simulink model "propeller_sim"  (R2022a)
settings: Solver=VariableStepAuto  StartTime=0.0  StopTime=10.0  MaxStep=0.02  RelTol=1e-3
values from neighbouring files (symbols this model uses):
  b = 1    [class8_PropellerPendulum.m]    (also in class8_PropellerPendulum_Euler.m = 0.1; class8_PropellerPendulum_ode45.m; epsac.m = 0.1; propeller.m = Par(4))
  g = 9.8    [class8_PropellerPendulum.m]    (also in class8_PropellerPendulum_Euler.m = 9.81; class8_PropellerPendulum_ode45.m; epsac.m = 9.81; propeller.m = Par(5))
  h = 0.5    [class8_PropellerPendulum.m]    (also in class8_PropellerPendulum_Euler.m; class8_PropellerPendulum_ode45.m; epsac.m; propeller.m = Par(1))
  Jeq = (M + m/3)*h^2    (= 0.0583333333333)    [class8_PropellerPendulum.m]    (also in class8_PropellerPendulum_Euler.m; class8_PropellerPendulum_ode45.m; epsac.m; propeller.m = Par(6))
  M = 0.1    [class8_PropellerPendulum.m]    (also in class8_PropellerPendulum_Euler.m; class8_PropellerPendulum_ode45.m; epsac.m; propeller.m = Par(2))
  m = 0.4    [class8_PropellerPendulum.m]    (also in class8_PropellerPendulum_Euler.m; class8_PropellerPendulum_ode45.m; epsac.m; propeller.m = Par(3))
settings Model: Creator=aaron  LastModifiedBy=aaron

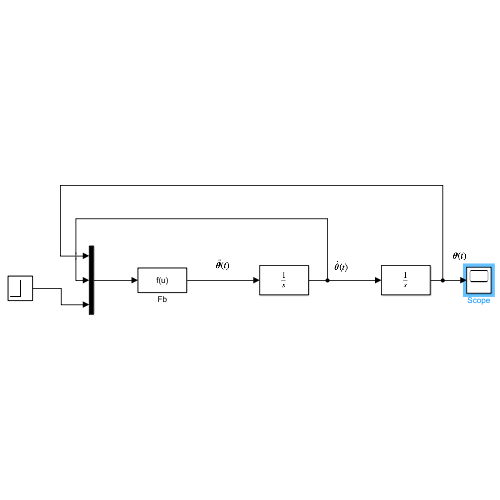
[thumbnail: Simulink's stored preview of the top-level diagram]
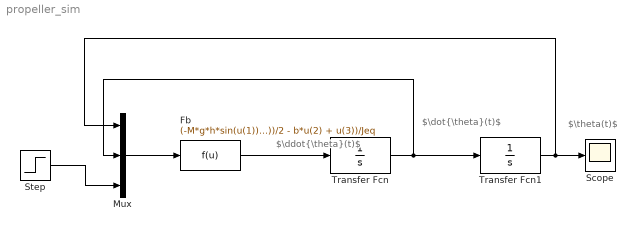
== system propeller_sim ==
  note: $\ddot{\theta}(t)$
  note: $\dot{\theta}(t)$
  note: $\theta(t)$
  Fb : Fcn  Expr=(-M*g*h*sin(u(1)) -m*g*h*sin(u(1))/2 - b*u(2) + u(3))/Jeq
  Mux : Mux  Inputs=3
  Scope : Scope
  Step : Step  Time=0  SampleTime=0
  Transfer Fcn : TransferFcn  Denominator=[1 0]
  Transfer Fcn1 : TransferFcn  Denominator=[1 0]
  wires:
  Fb/1 -> Transfer Fcn/1
  Transfer Fcn/1 -> Mux/2, Transfer Fcn1/1
  Transfer Fcn1/1 -> Scope/1, Mux/1
  Step/1 -> Mux/3
  Mux/1 -> Fb/1
